simulink model "ecal_helloworld_rec"  (R2021a)
settings: Solver=FixedStepDiscrete  StartTime=0.0  StopTime=inf  RelTol=1e-3
undefined symbols (not defined in the file): base, std
libraries: eCAL_blks_lib x1
settings Model: EnablePacing=on  Creator=uidp3321  LastModifiedBy=promero
settings SolverCC: ConcurrentTasks=on  AlgebraicLoopSolver=TrustRegion  PositivePriorityOrder=on
settings DataIOCC: ReturnWorkspaceOutputs=off
settings OptimizationCC: BlockReduction=off  OptimizeBlockIOStorage=off
settings DebuggingCC: TasksWithSamePriorityMsg=none  SFMachineParentedDataDiag=warning  ArithmeticOperatorsInVariantConditions=warning
settings HardwareCC: ProdBitPerLong=64  ProdLongLongMode=on  ProdHWDeviceType=Intel->x86-64 (Linux 64)
settings SFSimCC: SimUseLocalCustomCode=off  CustomCodeUndefinedFunction=UseInterfaceOnly  SimTargetLang=C++
settings RTWCC: Description=Simulink Real-Time  SystemTargetFile=slrealtime.tlc  TemplateMakefile=slrealtime_default_tmf  RTWUseLocalCustomCode=off  Toolchain=Simulink Real-Time Toolchain  BuildConfiguration=Faster Runs  CodeExecutionProfiling=on  TargetLang=C++
settings SimulinkRealTimeTargetCC: UseGCCFastMath=on

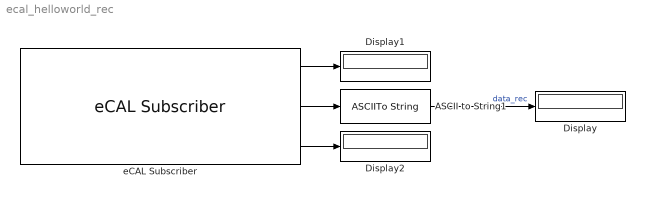
== system ecal_helloworld_rec ==
  ASCII to String1 : ASCIIToString
  Display : Display
  Display1 : Display
  Display2 : Display
  eCAL Subscriber : eCAL_blks_lib/eCAL Subscriber  param_topic_name=Hello  param_topic_type=base:std::string  param_max_buffer_size=50  param_signal_type=fixed  param_sample_time=0.25
      settings: SourceProductName=eCAL Blockset
  wires:
  eCAL Subscriber/2 -> ASCII to String1/1
  ASCII to String1/1 -> Display/1  "data_rec"
  eCAL Subscriber/1 -> Display1/1
  eCAL Subscriber/3 -> Display2/1
